simulink model "UdpImuSocket_Example"  (R2013a)
settings: Solver=ode45  StartTime=0.0  StopTime=inf  RelTol=1e-3
settings Model: Creator=jsUni  LastModifiedBy=jsUni

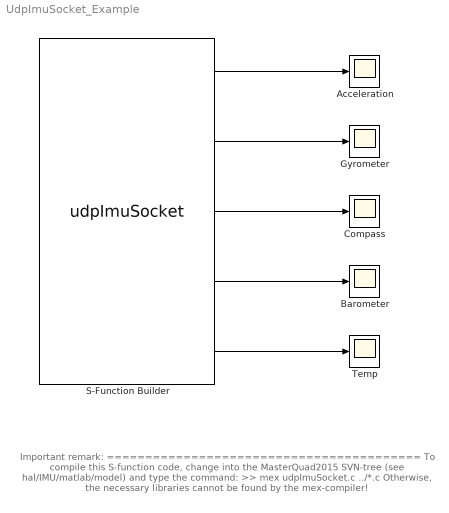
== system UdpImuSocket_Example ==
  note: Important remark:
      | =========================================
      |  To compile this S-function code, change into the MasterQuad2015
      | SVN-tree (see hal/IMU/matlab/model) and type the command:
      | >> mex udpImuSocket.c ../*.c
      |
      | Otherwise, the necessary libraries cannot be found by the mex-compiler!
  Acceleration : Scope
      settings: YMin=-45  YMax=10
  Barometer : Scope
      settings: YMin=976.55  YMax=977.2  SaveName=ScopeData3
  Compass : Scope
      settings: YMin=-5e-06  YMax=2.5e-05  SaveName=ScopeData2
  Gyrometer : Scope
      settings: YMin=-550  YMax=500
  S-Function Builder : S-Function  InitFcn=try, set_param(gcb,'FunctionName','udpImuSocket'), end  FunctionName=udpImuSocket  Parameters=0.02,5000  SFunctionModules=udpImuSocket_wrapper  EnableBusSupport=off  mask(S-Function Builder){}
      mask help: Simulink:masks:SFunctionBuilder_MD
      mask init:
      | val = [[.9  0.75 0.75 1 1 .9 .9 1]',[1 1 0.75 0.75 .9 .9 1 .9]'];try , sys = get_param(gcb,'SfunBuilderFcnName');if isempty(sys), sys = get_param(gcb,'FunctionName'); end,catch, sys = get_param(gcb,'FunctionName'); end
      settings: CopyFcn=set_param(gcbh,'LinkStatus','none')  PreSaveFcn=try, set_param(gcb,'FunctionName','udpImuSocket'), end  OpenFcn=sfunctionwizard(gcbh)
      mask Display: plot(val(:,1),val(:,2)),disp(sys), port_label('output',1,'Accelerometer'), port_label('output',2,'Gyrometer'), port_label('output',3,'Compass'), port_label('output',4,'Barometer'), port_label('output',5,'Temperature')
  Temp : Scope
      settings: YMin=32.2  YMax=32.29  SaveName=ScopeData4
  wires:
  S-Function Builder/3 -> Compass/1
  S-Function Builder/2 -> Gyrometer/1
  S-Function Builder/1 -> Acceleration/1
  S-Function Builder/5 -> Temp/1
  S-Function Builder/4 -> Barometer/1
